simulink model "Task2"  (R2022a)
settings: Solver=VariableStepAuto  StartTime=0.0  StopTime=10  RelTol=1e-3
settings Model: Creator=Family  LastModifiedBy=Family

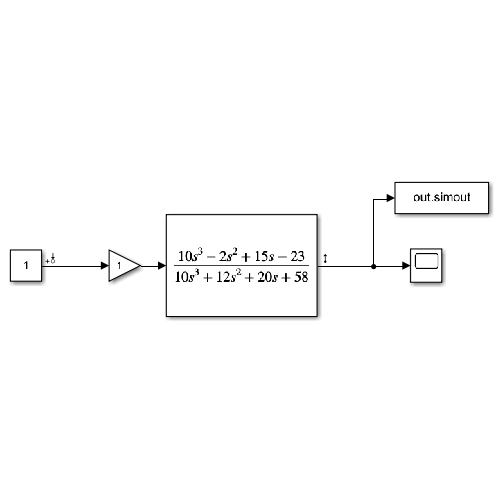
[thumbnail: Simulink's stored preview of the top-level diagram]
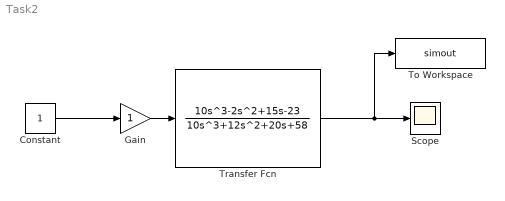
== system Task2 ==
  Constant : Constant  SampleTime=-1
  Gain : Gain
  Scope : Scope
  To Workspace : ToWorkspace  VariableName=simout  SaveFormat=Timeseries  SampleTime=-1
  Transfer Fcn : TransferFcn  Numerator=[10 -2 15 -23]  Denominator=[10 12 20 58]
  wires:
  Gain/1 -> Transfer Fcn/1
  Constant/1 -> Gain/1
  Transfer Fcn/1 -> To Workspace/1, Scope/1
